simulink subsystem "MotoresHF"  (R2023b)
settings: Solver=VariableStepAuto  StartTime=0.0  StopTime=10.0  RelTol=1e-3
libraries: arduinolib x6
settings Model: Creator=Hajar  LastModifiedBy=Hajar

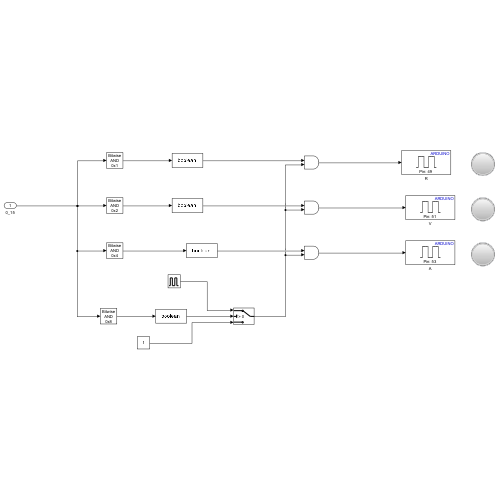
[thumbnail: Simulink's stored preview of the top-level diagram]
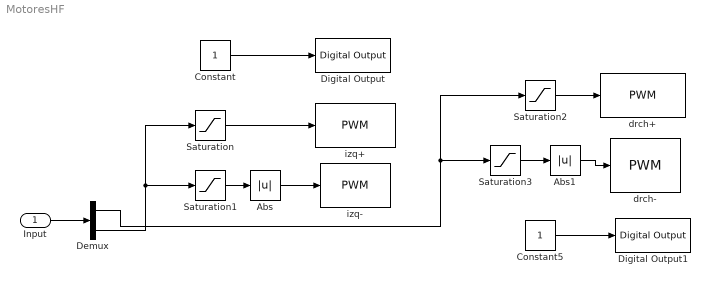
== system MotoresHF ==
  Input : Inport
  Abs : Abs  SaturateOnIntegerOverflow=off
  Abs1 : Abs  SaturateOnIntegerOverflow=off
  Constant : Constant
  Constant5 : Constant
  Demux : Demux  Outputs=2
  Digital Output : arduinolib/Digital Output  pinNumber=8  Direction=output  blockPlatform=arduino
  Digital Output1 : arduinolib/Digital Output  pinNumber=13  Direction=output  blockPlatform=arduino
  Saturation : Saturate  UpperLimit=+255  LowerLimit=0
  Saturation1 : Saturate  UpperLimit=0  LowerLimit=-255
  Saturation2 : Saturate  UpperLimit=+255  LowerLimit=0
  Saturation3 : Saturate  UpperLimit=0  LowerLimit=-255
  drch+ : arduinolib/PWM  pinNumber=11  frequencyType=Default  desiredFrequency=490.2  achievableFrequency=490.2
  drch- : arduinolib/PWM  pinNumber=12  frequencyType=Default  desiredFrequency=490.2  achievableFrequency=490.2
  izq+ : arduinolib/PWM  pinNumber=10  frequencyType=Default  desiredFrequency=490.2  achievableFrequency=490.2
  izq- : arduinolib/PWM  pinNumber=9  frequencyType=Default  desiredFrequency=490.2  achievableFrequency=490.2
  wires:
  Abs/1 -> izq-/1
  Constant/1 -> Digital Output/1
  Input/1 -> Demux/1
  Saturation/1 -> izq+/1
  Abs1/1 -> drch-/1
  Saturation2/1 -> drch+/1
  Saturation1/1 -> Abs/1
  Saturation3/1 -> Abs1/1
  Constant5/1 -> Digital Output1/1
  Demux/2 -> Saturation1/1, Saturation/1
  Demux/1 -> Saturation3/1, Saturation2/1
